simulink model "DQ20140501026"  (R2015a)
settings: Solver=ode45  StartTime=0.0  StopTime=5  RelTol=1e-3
libraries: powerlib x12, powerlib_extras x3
settings Model: Creator=Administrator  LastModifiedBy=佳君
settings DataIOCC: SignalLoggingSaveFormat=ModelDataLogs
settings OptimizationCC: ExpressionDepthLimit=2147483647
settings DebuggingCC: UnderspecifiedInitializationDetection=Classic  MergeDetectMultiDrivingBlocksExec=none  SolverPrmCheckMsg=warning  FcnCallInpInsideContextMsg=UseLocalSettings  StateNameClashWarn=warning  StrictBusMsg=Warning
settings GRTTargetCC: CombineOutputUpdateFcns=off  GRTInterface=on

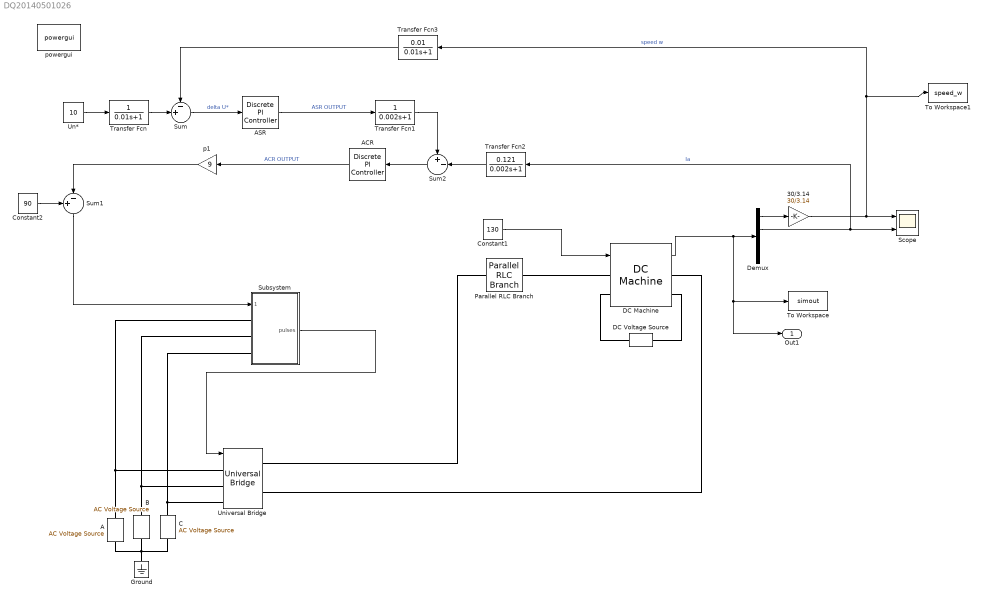
== system DQ20140501026 ==
  30/3.14 : Gain  Gain=30/3.14
  A : powerlib/Electrical Sources/AC Voltage Source  Amplitude=220  Phase=0  Frequency=50  SampleTime=0  Measurements=Voltage
  ACR : powerlib_extras/Discrete  Control Blocks/Discrete PI Controller  Kp=0.43  Ki=25.3  Par_Limits=[10 0]  Init=0  Ts=50e-6
  ASR : powerlib_extras/Discrete  Control Blocks/Discrete PI Controller  Kp=6.02  Ki=69.154  Par_Limits=[10 0]  Init=0  Ts=50e-6
  B : powerlib/Electrical Sources/AC Voltage Source  Amplitude=220  Phase=240  Frequency=50  SampleTime=0  Measurements=Voltage
  C : powerlib/Electrical Sources/AC Voltage Source  Amplitude=220  Phase=120  Frequency=50  SampleTime=0  Measurements=Voltage
  Constant1 : Constant  Value=130
  Constant2 : Constant  Value=90
  DC Machine : powerlib/Machines/DC Machine  PresetModel=No  MechanicalLoad=Torque TL  FieldType=Wound  ShowDetailedParameters=on  MeasurementBus=off  RLa=[0.5 0.017]  RLf=[240 120]  Laf=2  MachineConstant=Torque constant (N.m/A)  Ke=1.8  Kt=1.8  J=0.255  Bm=0  Tf=0  w0=1  Ifinit=0.916666666666667  TsPowergui=0  TsBlock=-1
  DC Voltage Source : powerlib/Electrical Sources/DC Voltage Source  Amplitude=220  Measurements=None
  Demux : Demux
  Ground : powerlib/Elements/Ground  LConnTagsString=a
  Parallel RLC Branch : powerlib/Elements/Parallel RLC Branch  LConnTagsString=a  RConnTagsString=__new0  BranchType=L  Resistance=1  Inductance=0.017  SetiL0=off  InitialCurrent=0  Capacitance=1e-6  Setx0=off  InitialVoltage=0  Measurements=Branch voltage and current
  Scope : Scope  NumInputPorts=2
      settings: TimeRange=5  YMin=-200~76.03286384976528  YMax=1200~79.08450704225355
  Subsystem : Subsystem
  Sum : Sum  Inputs=-+|
  Sum1 : Sum  Inputs=+-|
  Sum2 : Sum  Inputs=+-|
  To Workspace : ToWorkspace  VariableName=simout  SaveFormat=Structure  SampleTime=-1
  To Workspace1 : ToWorkspace  VariableName=speed_w  SaveFormat=Structure With Time  SampleTime=-1
  Transfer Fcn : TransferFcn  Denominator=[0.01 1]
  Transfer Fcn1 : TransferFcn  Denominator=[0.002 1]
  Transfer Fcn2 : TransferFcn  Numerator=0.121  Denominator=[0.002 1]
  Transfer Fcn3 : TransferFcn  Numerator=0.01  Denominator=[0.01 1]
  Un* : Constant  Value=10
  Universal Bridge : powerlib/Power Electronics/Universal Bridge  Arms=3  SnubberResistance=1e5  SnubberCapacitance=inf  Device=Thyristors  Ron=0.5  Lon=0  ForwardVoltages="[  0  0  ]"  ForwardVoltage=0  GTOparameters=[ 10e-6 , 20e-6 ]  IGBTparameters=[ 1e-6 , 2e-6 ]  Measurements=None  Measurements_2=None  converterType=Rectifier
  p1 : Gain  Gain=9
  powergui : powerlib/powergui  Priority=1  SimulationMode=Continuous  SolverType=Tustin/Backward Euler (TBE)  SampleTime=50e-6  frequency=60  SPID=off  DisableSnubberDevices=off  DisableRonSwitches=off  DisableVfSwitches=off  SwTol=0  DisplayEquations=off  Interpol=off  methode=off  Ts=0  FunctionMessages=off  echomessages=off  HookPort=off  EnableUseOfTLC=off  x0status=blocks  frequencyindice=0  Pbase=100e6  ErrMax=1e-4  Iterations=50  UnitsV=kV  UnitsW=MW  buscounter=0  RestoreLinks=warning  ResistiveCurrentMeasurement=off  Frange=[0:2:500]  Ylog=off  Xlog=on  ShowGrid=off  save=off  variable=ZData  structure=0  ZoomFFT=on  StartTime=0.0  cycles=1  DisplayStyle=1  fundamental=60  FreqAxis=off  MaxFrequency=1000  frequencyindicesteady=1  RmsSteady=1  display=off
  Out1 : Outport
  wires:
  DC Machine/1 -> Demux/1, Out1/1, To Workspace/1
  Demux/2 -> Transfer Fcn2/1, Scope/2  "Ia"
  Demux/1 -> 30/3.14/1
  Un*/1 -> Transfer Fcn/1
  30/3.14/1 -> To Workspace1/1, Transfer Fcn3/1, Scope/1  "speed w"
  Transfer Fcn3/1 -> Sum/1
  Sum/1 -> ASR/1  "delta U*"
  p1/1 -> Sum1/2
  Constant2/1 -> Sum1/1
  Sum1/1 -> Subsystem/1(alpha_deg)
  Constant1/1 -> DC Machine/1
  Transfer Fcn/1 -> Sum/2
  Sum2/1 -> ACR/1
  Transfer Fcn1/1 -> Sum2/1
  Transfer Fcn2/1 -> Sum2/2
  ACR/1 -> p1/1  "ACR OUTPUT"
  ASR/1 -> Transfer Fcn1/1  "ASR OUTPUT"
  Subsystem/1(pulses) -> Universal Bridge/1
  connections:
  Parallel RLC Branch/LConn1 -- Universal Bridge/RConn1
  DC Machine/RConn2 -- DC Voltage Source/LConn1
  DC Machine/LConn2 -- DC Voltage Source/RConn1
  Universal Bridge/RConn2 -- DC Machine/RConn1
  Parallel RLC Branch/RConn1 -- DC Machine/LConn1
  Ground/LConn1 -- A/LConn1 -- C/LConn1 -- B/LConn1
  Universal Bridge/LConn1 -- Subsystem/LConn1 -- A/RConn1
  Universal Bridge/LConn2 -- B/RConn1 -- Subsystem/LConn2
  Universal Bridge/LConn3 -- C/RConn1 -- Subsystem/LConn3

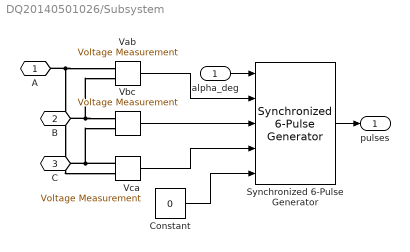
== system DQ20140501026/Subsystem ==
  alpha_deg : Inport
  Constant : Constant  Value=0
  Synchronized 6-Pulse Generator : powerlib_extras/Control  Blocks/Synchronized 6-Pulse Generator  freq=50  pwidth=10  Double_Pulse=off
  Vab : powerlib/Measurements/Voltage Measurement  PhasorSimulation=off  OutputType=Complex  PSBequivalent=0
  Vbc : powerlib/Measurements/Voltage Measurement  PhasorSimulation=off  OutputType=Complex  PSBequivalent=0
  Vca : powerlib/Measurements/Voltage Measurement  PhasorSimulation=off  OutputType=Complex  PSBequivalent=0
  A : PMIOPort  Port=1  Side=Left
  B : PMIOPort  Port=2  Side=Left
  C : PMIOPort  Port=3  Side=Left
  pulses : Outport
  wires:
  Vab/1 -> Synchronized 6-Pulse Generator/2
  Vbc/1 -> Synchronized 6-Pulse Generator/3
  Vca/1 -> Synchronized 6-Pulse Generator/4
  Constant/1 -> Synchronized 6-Pulse Generator/5
  alpha_deg/1 -> Synchronized 6-Pulse Generator/1
  Synchronized 6-Pulse Generator/1 -> pulses/1
  connections:
  A/RConn1 -- Vca/LConn2 -- Vab/LConn1
  B/RConn1 -- Vbc/LConn1 -- Vab/LConn2
  C/RConn1 -- Vca/LConn1 -- Vbc/LConn2
